simulink model "mbd_three"  (R2020b)
settings: Solver=VariableStepAuto  StartTime=0.0  StopTime=10.0  RelTol=1e-3
settings Model: Creator=SHWETA  LastModifiedBy=SHWETA

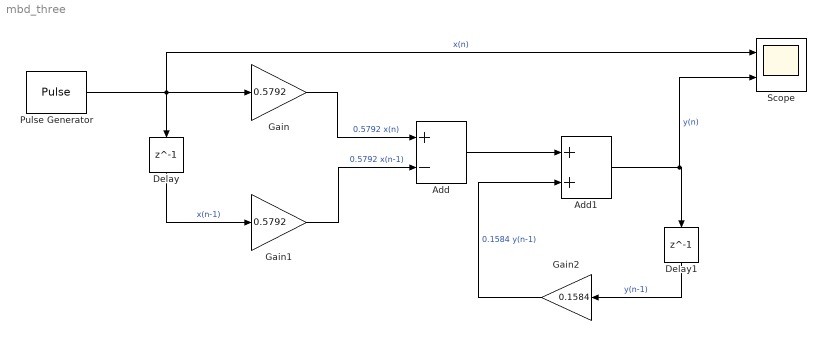
== system mbd_three ==
  Add : Sum  Inputs=+-
  Add1 : Sum
  Delay : Delay  DelayLength=1
  Delay1 : Delay  DelayLength=1
  Gain : Gain  Gain=0.5792
  Gain1 : Gain  Gain=0.5792
  Gain2 : Gain  Gain=0.1584
  Pulse Generator : DiscretePulseGenerator  PulseType=Time based  Period=10  PulseWidth=5
  Scope : Scope  NumInputPorts=2
  wires:
  Pulse Generator/1 -> Delay/1, Scope/1, Gain/1  "x(n)"
  Gain/1 -> Add/1  "0.5792 x(n)"
  Delay/1 -> Gain1/1  "x(n-1)"
  Gain1/1 -> Add/2  "0.5792 x(n-1)"
  Add/1 -> Add1/1
  Add1/1 -> Scope/2, Delay1/1  "y(n)"
  Delay1/1 -> Gain2/1  "y(n-1)"
  Gain2/1 -> Add1/2  "0.1584 y(n-1)"
